simulink model "cw5_model_Gajda"  (R2017b)
settings: Solver=VariableStepAuto  StartTime=0.0  StopTime=20.0  MaxStep=0.01  MinStep=0.001  RelTol=1e-6
values from neighbouring files (symbols this model uses):
  A = [-a0 a0; b0 (-b0-b1)]    [cw5_dane_Gajda.m]
  a0 = 1/(R1*C1)    (= 0.2)    [cw5_dane_Gajda.m]
  a1 = 1/C1    (= 0.1)    [cw5_dane_Gajda.m]
  B = [a1; 0]    [cw5_dane_Gajda.m]
  b0 = 1/(R1*C2)    (= 0.4)    [cw5_dane_Gajda.m]
  C = [0 1]    [cw5_dane_Gajda.m]
  D = [0]    [cw5_dane_Gajda.m]
settings Model: Creator=MG  LastModifiedBy=MG
settings DataIOCC: SaveFormat=Array

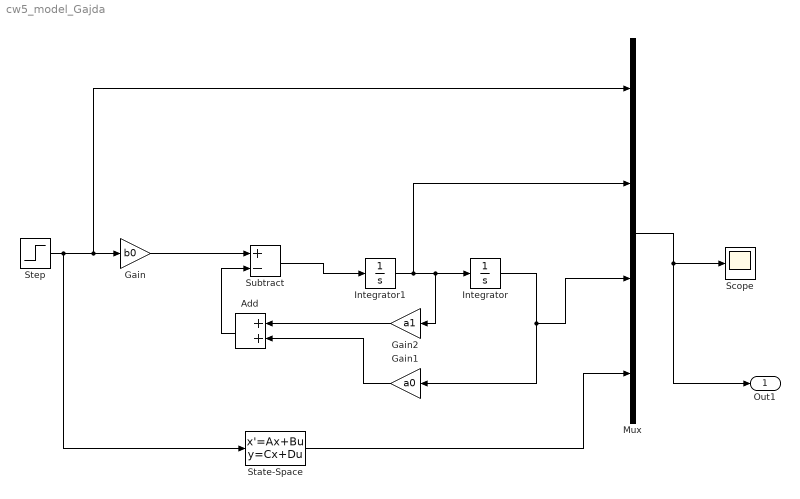
== system cw5_model_Gajda ==
  Add : Sum
  Gain : Gain  Gain=b0
  Gain1 : Gain  Gain=a0
  Gain2 : Gain  Gain=a1
  Integrator : Integrator
  Integrator1 : Integrator
  Mux : Mux
  Scope : Scope
  State-Space : StateSpace  A=A  B=B  C=C  D=D  InitialCondition=0
  Step : Step  Time=0  SampleTime=0
  Subtract : Sum  Inputs=+-
  Out1 : Outport
  wires:
  Gain2/1 -> Add/1
  Mux/1 -> Out1/1, Scope/1
  Add/1 -> Subtract/2
  Step/1 -> Gain/1, Mux/1, State-Space/1
  Integrator1/1 -> Mux/2, Gain2/1, Integrator/1
  Integrator/1 -> Gain1/1, Mux/3
  Subtract/1 -> Integrator1/1
  State-Space/1 -> Mux/4
  Gain/1 -> Subtract/1
  Gain1/1 -> Add/2
